simulink model "CSE1_HIL_full_Test"  (R2019b)
settings: Solver=VariableStepAuto  StartTime=0.0  StopTime=150  MaxStep=10e-3  RelTol=1e-3
values from neighbouring files (symbols this model uses):
  B = [zeros(3); inv(M); zeros(3)]    [CSE1_init.m]
  center_point = [0 0]'    [CSE1_init.m]
  D = [ ... (first row only)    [CSE1_init.m]    (also in D.m = reshape([abs(u).*(-3.545e-1)+u.^2.*3.787+6.555e-1,0.0,0.0,0.)
  end_point = [10 10]'    [CSE1_init.m]
  Kd = 1e-2    (= 0.01)    [CSE1_init.m]    (also in run.m = diag([40e-2 40e-2 40e-2]))
  Kp = 1e-2    (= 0.01)    [CSE1_init.m]    (also in run.m = diag([25e-2 25e-2 25e-4]))
  L1 = diag([1 1 1])    [CSE1_init.m]
  L2 = diag([0.1 0.1 0.1])    [CSE1_init.m]
  L3 = diag([0.025 0.01 0.0001])    [CSE1_init.m]
  M = [ ... (first row only)    [CSE1_init.m]
  measurement_signal_available = 1    [CSE1_init.m]
  measurment_noise = 0    [CSE1_init.m]
  my = 0.05    [CSE1_init.m]
  path_selection = 0    [CSE1_init.m]
  radius_xy = diag([1 2])    [CSE1_init.m]
  start_point = [0 0]'    [CSE1_init.m]
  U_ref = 0.15    [CSE1_init.m]
  x_init = zeros(1,9)    [CSE1_init.m]
libraries: simulink x1
settings Model: Creator=einarsu  LastModifiedBy=linnl
settings DataIOCC: ReturnWorkspaceOutputs=off
settings OptimizationCC: LifeSpan=inf
settings DebuggingCC: SFExecutionAtInitializationDiag=none  ArithmeticOperatorsInVariantConditions=warning
settings SFSimCC: SimUseLocalCustomCode=off  CustomCodeUndefinedFunction=UseInterfaceOnly
settings RTWCC: RTWUseLocalCustomCode=off
settings CodeAppCC: StateflowObjectComments=on

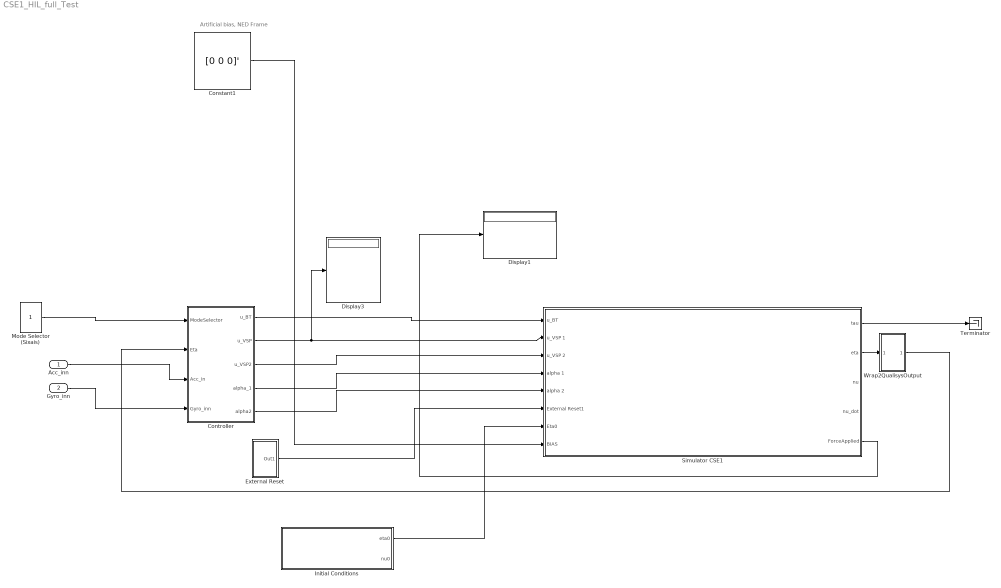
== system CSE1_HIL_full_Test ==
  note: Artificial bias, NED Frame
  Acc_inn : Inport
  Gyro_inn : Inport  Port=2
  Constant1 : Constant  Value=[0 0 0]'  VectorParams1D=off
  Controller : Subsystem
  Display1 : Display
  Display3 : Display
  External Reset : Subsystem
  "Initial Conditions " : Subsystem
  Mode Selector (Sixais) : Constant
  Simulator CSE1 : Subsystem
  Terminator : Terminator
  "Wrap2QualisysOutput " : Subsystem
  wires:
  Controller/1(u_BT) -> Simulator CSE1/1(u_BT)
  Controller/4(alpha_1) -> Simulator CSE1/4(alpha 1)
  Controller/2(u_VSP) -> Display3/1, Simulator CSE1/2(u_VSP 1)
  Controller/5(alpha2) -> Simulator CSE1/5(alpha 2)
  Controller/3("u_VSP2 ") -> Simulator CSE1/3(u_VSP 2)
  Simulator CSE1/1(tau) -> Terminator/1
  External Reset/1(Out1) -> Simulator CSE1/6(External Reset1)
  "Initial Conditions "/1(eta0) -> Simulator CSE1/7(Eta0)
  Mode Selector (Sixais)/1 -> Controller/1(ModeSelector)
  Simulator CSE1/2(eta) -> "Wrap2QualisysOutput "/1(In1)
  Acc_inn/1 -> Controller/3(Acc_in)
  Gyro_inn/1 -> Controller/4(Gyro_inn)
  Simulator CSE1/5(ForceApplied) -> Display1/1
  Constant1/1 -> Simulator CSE1/8(BIAS)
  "Wrap2QualisysOutput "/1(Out1) -> Controller/2(Eta)

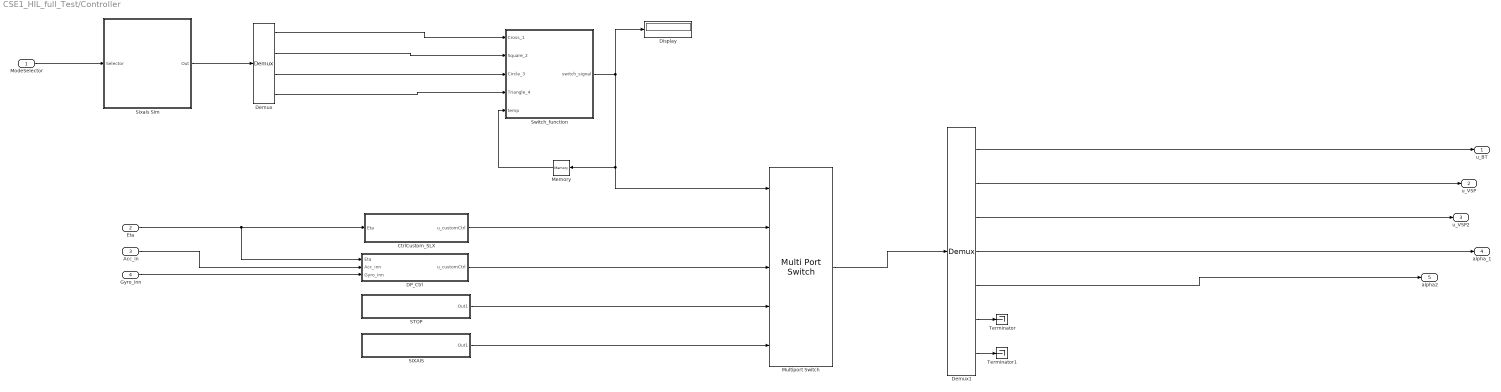
== system CSE1_HIL_full_Test/Controller ==
  ModeSelector : Inport
  Eta : Inport  Port=2
  Acc_in : Inport  Port=3
  Gyro_inn : Inport  Port=4
  CtrlCustom_SLX : Subsystem
  DP_Ctrl : Subsystem
  Demux : Demux
  Demux1 : Demux  Outputs=7
  Display : Display
  Memory : Memory  InitialCondition=4
  Multiport Switch : MultiPortSwitch  Inputs=4
  SIXAIS : Subsystem
  STOP : Subsystem
  Sixais Sim : MATLAB Function  TreatAsAtomicUnit=on
  Switch_function : MATLAB Function  TreatAsAtomicUnit=on
  Terminator : Terminator
  Terminator1 : Terminator
  u_BT : Outport
  u_VSP : Outport  Port=2
  "u_VSP2 " : Outport  Port=3
  alpha_1 : Outport  Port=4
  alpha2 : Outport  Port=5
  wires:
  Switch_function/1(switch_signal) -> Display/1, Memory/1, Multiport Switch/1
  Memory/1 -> Switch_function/5(temp)
  CtrlCustom_SLX/1(u_customCtrl) -> Multiport Switch/2
  Demux/1 -> Switch_function/1(Cross_1)
  Demux/2 -> Switch_function/2(Square_2)
  Demux/3 -> Switch_function/3(Circle_3)
  Demux/4 -> Switch_function/4(Triangle_4)
  Sixais Sim/1(Out) -> Demux/1
  ModeSelector/1 -> Sixais Sim/1(Selector)
  DP_Ctrl/1(u_customCtrl) -> Multiport Switch/3
  STOP/1(Out1) -> Multiport Switch/4
  SIXAIS/1(Out1) -> Multiport Switch/5
  Eta/1 -> CtrlCustom_SLX/1(Eta), DP_Ctrl/1(Eta)
  Acc_in/1 -> DP_Ctrl/2(Acc_inn)
  Gyro_inn/1 -> DP_Ctrl/3(Gyro_inn)
  Multiport Switch/1 -> Demux1/1
  Demux1/1 -> u_BT/1
  Demux1/2 -> u_VSP/1
  Demux1/3 -> "u_VSP2 "/1
  Demux1/4 -> alpha_1/1
  Demux1/5 -> alpha2/1
  Demux1/6 -> Terminator/1
  Demux1/7 -> Terminator1/1

== system CSE1_HIL_full_Test/External Reset ==
  note: Most relevant for Real-Time Simulations...
  Constant : Constant  Value=0
  Out1 : Outport
  wires:
  Constant/1 -> Out1/1

== system CSE1_HIL_full_Test/Initial Conditions  ==
  Eta0 : Constant  Value=zeros(3,1)
  "V0 " : Constant  Value=zeros(3,1)
  eta0 : Outport
  nu0 : Outport  Port=2
  wires:
  "V0 "/1 -> nu0/1
  Eta0/1 -> eta0/1

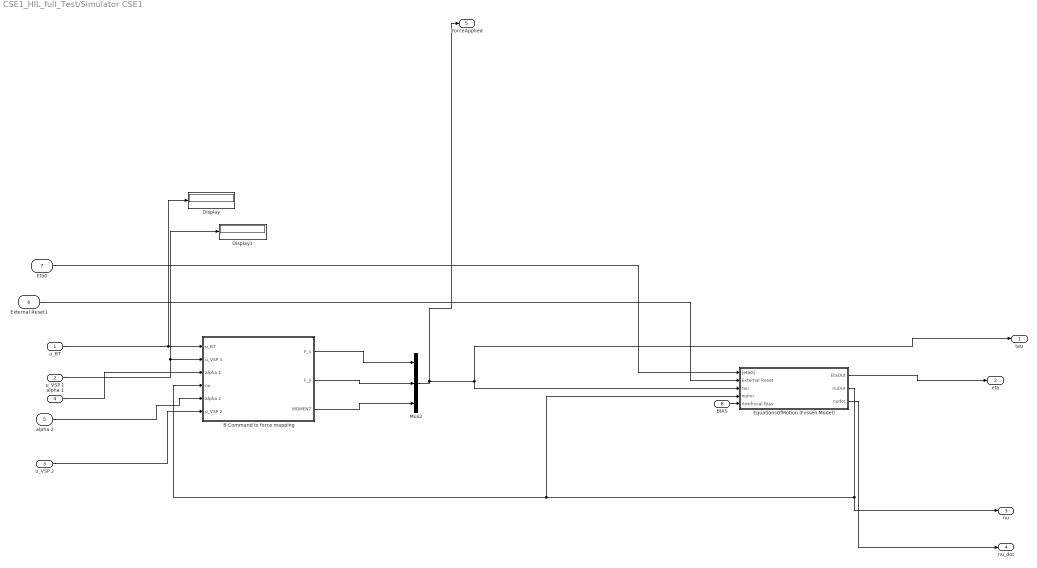
== system CSE1_HIL_full_Test/Simulator CSE1 ==
  u_BT : Inport
  u_VSP 1 : Inport  Port=2
  u_VSP 2 : Inport  Port=3
  alpha 1 : Inport  Port=4
  alpha 2 : Inport  Port=5
  External Reset1 : Inport  Port=6
  Eta0 : Inport  Port=7
  BIAS : Inport  Port=8
  B Command to force mapping : Subsystem
  Display : Display
  Display1 : Display
  EquationsOfMotion (Fossen Model) : Subsystem
  Mux2 : Mux  Inputs=3
  tau : Outport
  eta : Outport  Port=2
  nu : Outport  Port=3
  nu_dot : Outport  Port=4
  ForceApplied : Outport  Port=5
  wires:
  alpha 2/1 -> B Command to force mapping/5(alpha 2)
  B Command to force mapping/2("F_y ") -> Mux2/2
  B Command to force mapping/1(F_x) -> Mux2/1
  u_VSP 1/1 -> B Command to force mapping/2(u_VSP 1), Display1/1
  alpha 1/1 -> B Command to force mapping/3(alpha 1)
  u_BT/1 -> B Command to force mapping/1(u_BT), Display/1
  u_VSP 2/1 -> B Command to force mapping/6(u_VSP 2)
  EquationsOfMotion (Fossen Model)/2(nuOut) -> B Command to force mapping/4(nu), EquationsOfMotion (Fossen Model)/4(nuInn), nu/1
  Eta0/1 -> EquationsOfMotion (Fossen Model)/1("[eta0] ")
  External Reset1/1 -> EquationsOfMotion (Fossen Model)/2(External Reset)
  Mux2/1 -> ForceApplied/1, EquationsOfMotion (Fossen Model)/3(tau), tau/1
  EquationsOfMotion (Fossen Model)/1(EtaOut) -> eta/1
  EquationsOfMotion (Fossen Model)/3(nudot) -> nu_dot/1
  B Command to force mapping/3("MOMENT ") -> Mux2/3
  BIAS/1 -> EquationsOfMotion (Fossen Model)/5(Aritifiicial BIas)

== system CSE1_HIL_full_Test/Wrap2QualisysOutput  ==
  In1 : Inport
  Demux : Demux  Outputs=3
  Gain : Gain  Gain=1000
  Gain1 : Gain  Gain=1000
  Gain2 : Gain  Gain=180/pi
  Mux : Mux  Inputs=3
  Wrap2psi : MATLAB Function  TreatAsAtomicUnit=on
  Out1 : Outport
  wires:
  Mux/1 -> Out1/1
  In1/1 -> Demux/1
  Demux/3 -> Wrap2psi/1(u)
  Demux/1 -> Gain/1
  Demux/2 -> Gain1/1
  Gain/1 -> Mux/1
  Gain1/1 -> Mux/2
  Gain2/1 -> Mux/3
  Wrap2psi/1(yQualisus) -> Gain2/1

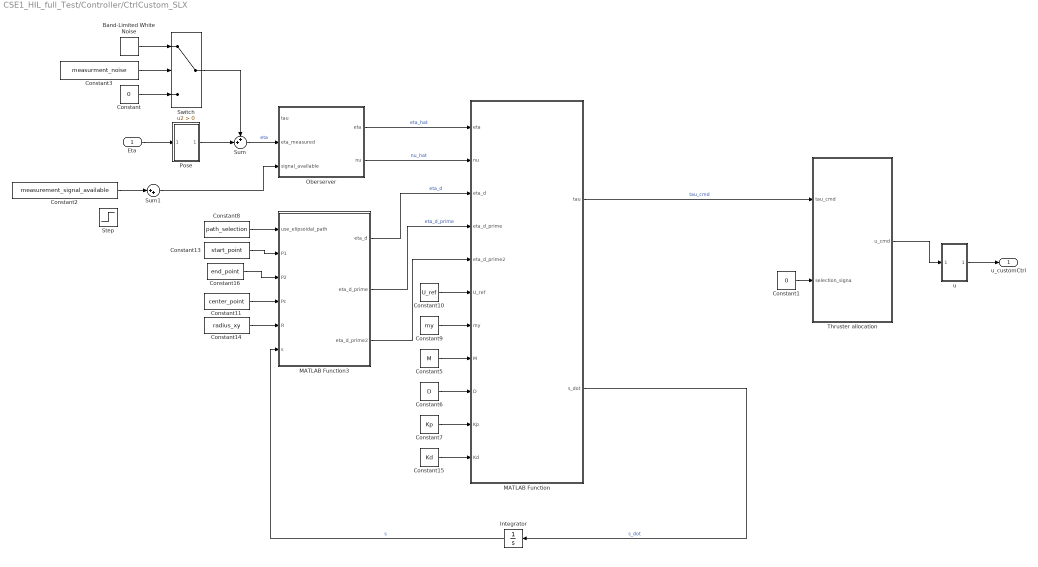
== system CSE1_HIL_full_Test/Controller/CtrlCustom_SLX ==
  Eta : Inport
  Band-Limited White Noise : simulink/Sources/Band-Limited White Noise  Cov=[0.01 0.01 0.001]'  Ts=0.1  seed=[23341]  VectorParams1D=off
  Constant : Constant  Value=0
  Constant1 : Constant  Value=0
  Constant10 : Constant  Value=U_ref
  Constant11 : Constant  Value=center_point
  Constant13 : Constant  Value=start_point
  Constant14 : Constant  Value=radius_xy
  Constant15 : Constant  Value=Kd
  Constant16 : Constant  Value=end_point
  Constant2 : Constant  Value=measurement_signal_available
  Constant3 : Constant  Value=measurment_noise
  Constant5 : Constant  Value=M
  Constant6 : Constant  Value=D
  Constant7 : Constant  Value=Kp
  Constant8 : Constant  Value=path_selection
  Constant9 : Constant  Value=my
  Integrator : Integrator
  MATLAB Function : MATLAB Function  TreatAsAtomicUnit=on
  MATLAB Function3 : MATLAB Function  TreatAsAtomicUnit=on
  Oberserver : Subsystem
  Pose : Subsystem
  Step : Step  Time=50  After=-1  SampleTime=0
  Sum : Sum  Inputs=++|
  Sum1 : Sum  Inputs=|++
  Switch : Switch  Criteria=u2 > Threshold
  Thruster allocation : Subsystem
  u : Subsystem
  u_customCtrl : Outport
  wires:
  Constant16/1 -> MATLAB Function3/3(P2)
  Constant14/1 -> MATLAB Function3/5(R)
  Constant15/1 -> MATLAB Function/11(Kd)
  Constant13/1 -> MATLAB Function3/2(P1)
  Oberserver/1(eta) -> MATLAB Function/1(eta)  "eta_hat"
  Eta/1 -> Pose/1(eta)
  Constant7/1 -> MATLAB Function/10(Kp)
  Thruster allocation/1(u_cmd) -> u/1(In1)
  Constant/1 -> Switch/3
  Constant1/1 -> Thruster allocation/2(selection_signa)
  u/1(Out1) -> u_customCtrl/1
  Constant10/1 -> MATLAB Function/6(U_ref)
  MATLAB Function3/3(eta_d_prime2) -> MATLAB Function/5(eta_d_prime2)
  Oberserver/2(nu) -> MATLAB Function/2(nu)  "nu_hat"
  MATLAB Function3/2(eta_d_prime) -> MATLAB Function/4(eta_d_prime)  "eta_d_prime"
  Sum1/1 -> Oberserver/3(signal_available)
  Constant9/1 -> MATLAB Function/7(my)
  Pose/1(QTM) -> Sum/2
  Constant2/1 -> Sum1/1
  MATLAB Function3/1(eta_d) -> MATLAB Function/3(eta_d)  "eta_d"
  Constant8/1 -> MATLAB Function3/1(use_elipsoidal_path)
  Band-Limited White Noise/1 -> Switch/1
  Sum/1 -> Oberserver/2(eta_measured)  "eta"
  Switch/1 -> Sum/1
  MATLAB Function/2(s_dot) -> Integrator/1  "s_dot"
  Constant11/1 -> MATLAB Function3/4(Pc)
  Constant5/1 -> MATLAB Function/8(M)
  Constant3/1 -> Switch/2
  Integrator/1 -> MATLAB Function3/6(s)  "s"
  MATLAB Function/1(tau) -> Thruster allocation/1(tau_cmd)  "tau_cmd"
  Constant6/1 -> MATLAB Function/9(D)

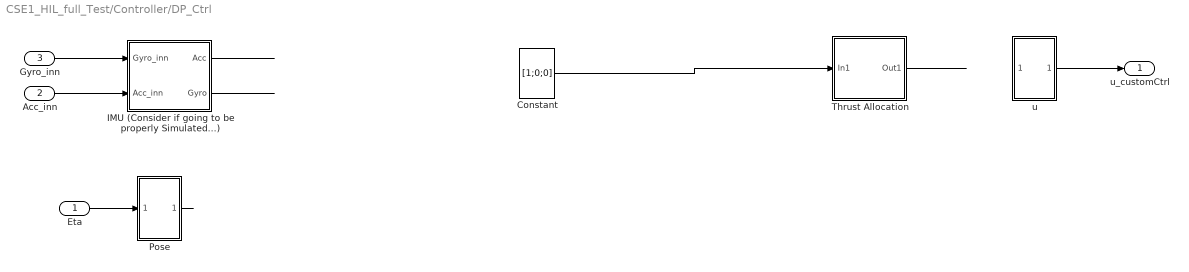
== system CSE1_HIL_full_Test/Controller/DP_Ctrl ==
  Eta : Inport
  Acc_inn : Inport  Port=2
  Gyro_inn : Inport  Port=3
  Constant : Constant  Value=[1;0;0]
  IMU (Consider if going to be properly Simulated...) : Subsystem
  Pose : Subsystem
  "Thrust Allocation " : Subsystem
  u : Subsystem
  u_customCtrl : Outport
  wires:
  Pose/1(QTM) -> ?
  Gyro_inn/1 -> IMU (Consider if going to be properly Simulated...)/1(Gyro_inn)
  Acc_inn/1 -> IMU (Consider if going to be properly Simulated...)/2(Acc_inn)
  Eta/1 -> Pose/1(eta)
  u/1(Out1) -> u_customCtrl/1
  IMU (Consider if going to be properly Simulated...)/2(Gyro) -> ?
  IMU (Consider if going to be properly Simulated...)/1(Acc) -> ?
  Constant/1 -> "Thrust Allocation "/1(In1)
  "Thrust Allocation "/1(Out1) -> ?

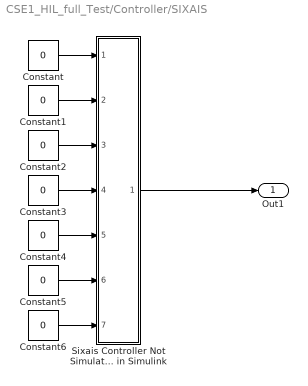
== system CSE1_HIL_full_Test/Controller/SIXAIS ==
  Constant{,1..6} (7 alike) : Constant  Value=0
  Sixais Controller Not Simulated in Simulink : Subsystem
  Out1 : Outport
  wires:
  Constant/1 -> Sixais Controller Not Simulated in Simulink/1(In1)
  Constant1/1 -> Sixais Controller Not Simulated in Simulink/2(In2)
  Constant2/1 -> Sixais Controller Not Simulated in Simulink/3(In3)
  Constant3/1 -> Sixais Controller Not Simulated in Simulink/4(In4)
  Constant4/1 -> Sixais Controller Not Simulated in Simulink/5(In5)
  Constant5/1 -> Sixais Controller Not Simulated in Simulink/6(In6)
  Constant6/1 -> Sixais Controller Not Simulated in Simulink/7(In7)
  Sixais Controller Not Simulated in Simulink/1(Out1) -> Out1/1

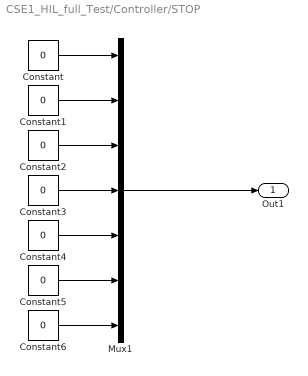
== system CSE1_HIL_full_Test/Controller/STOP ==
  Constant{,1..6} (7 alike) : Constant  Value=0
  Mux1 : Mux  Inputs=7
  Out1 : Outport
  wires:
  Mux1/1 -> Out1/1
  Constant/1 -> Mux1/1
  Constant1/1 -> Mux1/2
  Constant2/1 -> Mux1/3
  Constant3/1 -> Mux1/4
  Constant4/1 -> Mux1/5
  Constant5/1 -> Mux1/6
  Constant6/1 -> Mux1/7

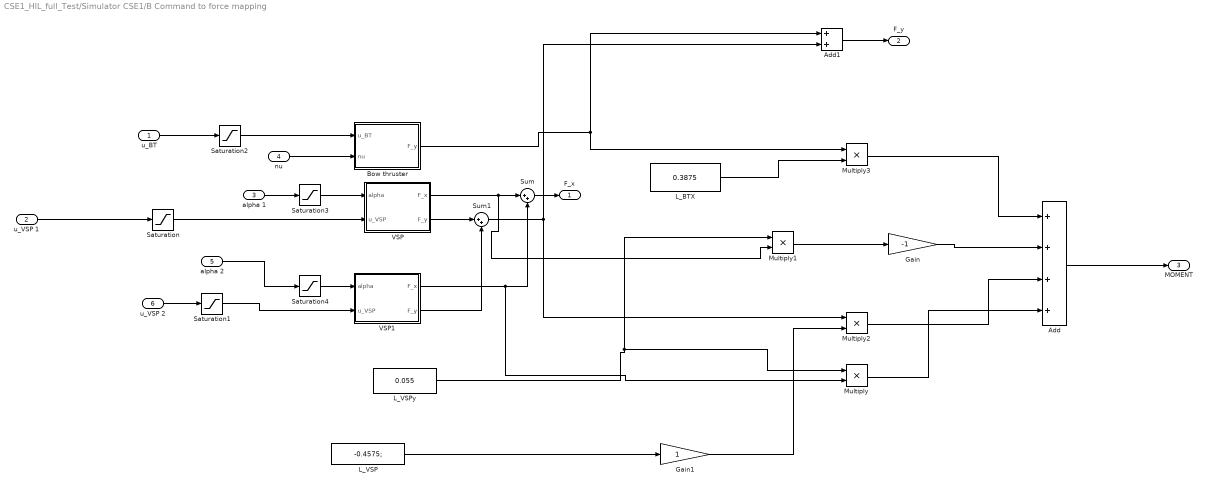
== system CSE1_HIL_full_Test/Simulator CSE1/B Command to force mapping ==
  u_BT : Inport
  u_VSP 1 : Inport  Port=2
  alpha 1 : Inport  Port=3
  nu : Inport  Port=4
  alpha 2 : Inport  Port=5
  u_VSP 2 : Inport  Port=6
  Add : Sum  Inputs=++++
  Add1 : Sum
  Bow thruster : MATLAB Function  TreatAsAtomicUnit=on
  Gain : Gain  Gain=-1
  Gain1 : Gain
  L_BTX : Constant  Value=0.3875
  L_VSP : Constant  Value=-0.4575;
  L_VSPy : Constant  Value=0.055
  Multiply{,1..3} (4 alike) : Product
  Saturation : Saturate  UpperLimit=1  LowerLimit=0
  Saturation1 : Saturate  UpperLimit=1  LowerLimit=0
  Saturation2 : Saturate  UpperLimit=1  LowerLimit=-1
  Saturation3 : Saturate  UpperLimit=pi  LowerLimit=-pi
  Saturation4 : Saturate  UpperLimit=pi  LowerLimit=-pi
  Sum : Sum  Inputs=|++
  Sum1 : Sum  Inputs=|++
  VSP : MATLAB Function  TreatAsAtomicUnit=on
  VSP1 : MATLAB Function  TreatAsAtomicUnit=on
  F_x : Outport
  "F_y " : Outport  Port=2
  "MOMENT " : Outport  Port=3
  wires:
  alpha 1/1 -> Saturation3/1
  nu/1 -> Bow thruster/2(nu)
  Bow thruster/1(F_y) -> Add1/1, Multiply3/1
  VSP/2(F_y) -> Sum1/1
  Sum1/1 -> Add1/2, Multiply2/1
  VSP1/2(F_y) -> Sum1/2
  VSP1/1(F_x) -> Multiply/2, Sum/2
  VSP/1(F_x) -> Multiply1/2, Sum/1
  Sum/1 -> F_x/1
  alpha 2/1 -> Saturation4/1
  u_VSP 2/1 -> Saturation1/1
  L_VSP/1 -> Gain1/1
  L_BTX/1 -> Multiply3/2
  L_VSPy/1 -> Multiply/1, Multiply1/1
  Multiply3/1 -> Add/1
  Multiply1/1 -> Gain/1
  Multiply2/1 -> Add/3
  Multiply/1 -> Add/4
  Add/1 -> "MOMENT "/1
  Gain/1 -> Add/2
  Gain1/1 -> Multiply2/2
  Add1/1 -> "F_y "/1
  Saturation/1 -> VSP/2(u_VSP)
  Saturation1/1 -> VSP1/2(u_VSP)
  u_BT/1 -> Saturation2/1
  u_VSP 1/1 -> Saturation/1
  Saturation2/1 -> Bow thruster/1(u_BT)
  Saturation3/1 -> VSP/1(alpha)
  Saturation4/1 -> VSP1/1(alpha)

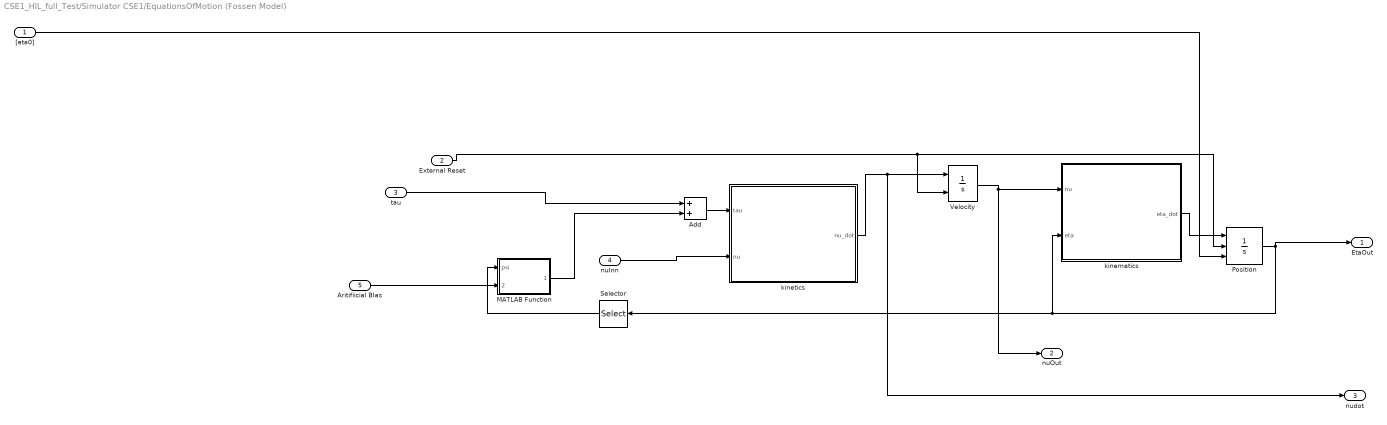
== system CSE1_HIL_full_Test/Simulator CSE1/EquationsOfMotion (Fossen Model) ==
  "[eta0] " : Inport
  External Reset : Inport  Port=2
  tau : Inport  Port=3
  nuInn : Inport  Port=4
  Aritifiicial BIas : Inport  Port=5
  Add : Sum
  MATLAB Function : MATLAB Function  TreatAsAtomicUnit=on
  Position : Integrator  ExternalReset=either  InitialConditionSource=external  InitialCondition=[0 0 0]'
  Selector : Selector  InputPortWidth=3  IndexOptions=Index vector (dialog)  Indices=[3]  OutputSizes=1
  Velocity : Integrator  ExternalReset=either  InitialCondition=[0 0 0]'
  kinematics : MATLAB Function  TreatAsAtomicUnit=on
  kinetics : MATLAB Function  TreatAsAtomicUnit=on
  EtaOut : Outport
  nuOut : Outport  Port=2
  nudot : Outport  Port=3
  wires:
  tau/1 -> Add/1
  Position/1 -> Selector/1, kinematics/2(eta), EtaOut/1
  "[eta0] "/1 -> Position/3
  nuInn/1 -> kinetics/2(nu)
  kinematics/1(eta_dot) -> Position/1
  Velocity/1 -> nuOut/1, kinematics/1(nu)
  kinetics/1(nu_dot) -> nudot/1, Velocity/1
  External Reset/1 -> Velocity/2, Position/2
  Add/1 -> kinetics/1(tau)
  Aritifiicial BIas/1 -> MATLAB Function/2(NedVector)
  Selector/1 -> MATLAB Function/1(psi)
  MATLAB Function/1(BodyVector) -> Add/2

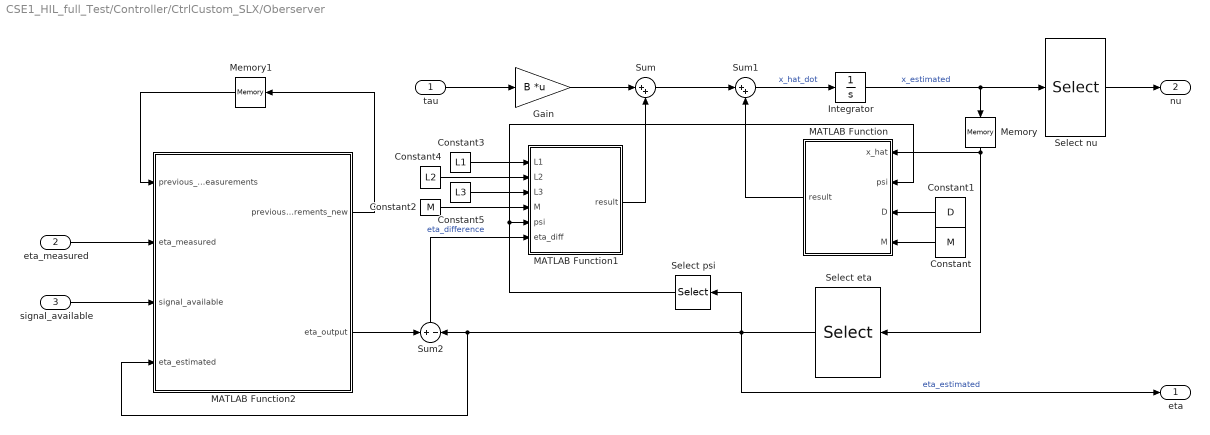
== system CSE1_HIL_full_Test/Controller/CtrlCustom_SLX/Oberserver ==
  tau : Inport
  eta_measured : Inport  Port=2
  signal_available : Inport  Port=3
  Constant : Constant  Value=M
  Constant1 : Constant  Value=D
  Constant2 : Constant  Value=M
  Constant3 : Constant  Value=L1
  Constant4 : Constant  Value=L2
  Constant5 : Constant  Value=L3
  Gain : Gain  Gain=B  Multiplication=Matrix(K*u) (u vector)
  Integrator : Integrator  InitialCondition=x_init
  MATLAB Function : MATLAB Function  TreatAsAtomicUnit=on
  MATLAB Function1 : MATLAB Function  TreatAsAtomicUnit=on
  MATLAB Function2 : MATLAB Function  TreatAsAtomicUnit=on
  Memory : Memory  InitialCondition=x_init
  Memory1 : Memory  InitialCondition=[0,0,0; 0,0,0; 0,0,0]
  Select eta : Selector  InputPortWidth=9  IndexOptions=Index vector (dialog)  Indices=[1 2 3]  OutputSizes=1
  Select nu : Selector  InputPortWidth=9  IndexOptions=Index vector (dialog)  Indices=[4 5 6]  OutputSizes=1
  Select psi : Selector  InputPortWidth=3  IndexOptions=Index vector (dialog)  Indices=[3]  OutputSizes=1
  Sum : Sum  Inputs=|++
  Sum1 : Sum  Inputs=|++
  Sum2 : Sum  Inputs=+|-
  eta : Outport
  nu : Outport  Port=2
  wires:
  Integrator/1 -> Select nu/1, Memory/1  "x_estimated"
  tau/1 -> Gain/1
  Gain/1 -> Sum/1
  Sum1/1 -> Integrator/1  "x_hat_dot"
  Sum/1 -> Sum1/1
  eta_measured/1 -> MATLAB Function2/2(eta_measured)
  MATLAB Function1/1(result) -> Sum/2
  MATLAB Function/1(result) -> Sum1/2
  Constant/1 -> MATLAB Function/4(M)
  Constant1/1 -> MATLAB Function/3(D)
  Memory/1 -> Select eta/1, MATLAB Function/1(x_hat)
  Select eta/1 -> MATLAB Function2/4(eta_estimated), Sum2/2, Select psi/1, eta/1  "eta_estimated"
  Constant2/1 -> MATLAB Function1/4(M)
  Constant3/1 -> MATLAB Function1/1(L1)
  Constant4/1 -> MATLAB Function1/2(L2)
  Constant5/1 -> MATLAB Function1/3(L3)
  signal_available/1 -> MATLAB Function2/3(signal_available)
  MATLAB Function2/1(previous_measurements_new) -> Memory1/1
  Memory1/1 -> MATLAB Function2/1(previous_measurements)
  Select nu/1 -> nu/1
  MATLAB Function2/2(eta_output) -> Sum2/1
  Sum2/1 -> MATLAB Function1/6(eta_diff)  "eta_difference"
  Select psi/1 -> MATLAB Function/2(psi), MATLAB Function1/5(psi)

== system CSE1_HIL_full_Test/Controller/CtrlCustom_SLX/Pose ==
  eta : Inport
  Demux : Demux  Outputs=3
  Gain : Gain  Gain=10^-3
  Gain1 : Gain  Gain=10^-3
  MATLAB Function : MATLAB Function  TreatAsAtomicUnit=on
  Mux : Mux  Inputs=3
  QTM : Outport
  wires:
  Demux/2 -> Gain1/1  "y_mm"
  Demux/3 -> MATLAB Function/1(deg)  "psi_deg"
  Mux/1 -> QTM/1
  eta/1 -> Demux/1
  Demux/1 -> Gain/1  "x_mm"
  Gain/1 -> Mux/1  "x_m"
  Gain1/1 -> Mux/2  "y_m"
  MATLAB Function/1(rad) -> Mux/3  "psi_rad"

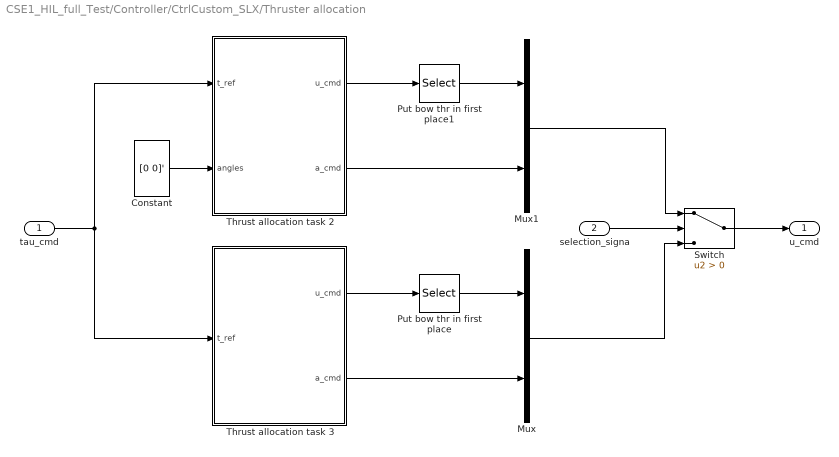
== system CSE1_HIL_full_Test/Controller/CtrlCustom_SLX/Thruster allocation ==
  tau_cmd : Inport
  selection_signa : Inport  Port=2
  Constant : Constant  Value=[0 0]'  VectorParams1D=off
  Mux : Mux  Inputs=2
  Mux1 : Mux  Inputs=2
  Put bow thr in first place : Selector  InputPortWidth=3  IndexOptions=Index vector (dialog)  Indices=[3 1 2]  OutputSizes=1
  Put bow thr in first place1 : Selector  InputPortWidth=3  IndexOptions=Index vector (dialog)  Indices=[3 1 2]  OutputSizes=1
  Switch : Switch  Criteria=u2 > Threshold
  Thrust allocation task 2 : Subsystem
  Thrust allocation task 3 : Subsystem
  u_cmd : Outport
  wires:
  Switch/1 -> u_cmd/1
  Constant/1 -> Thrust allocation task 2/2(angles)
  Thrust allocation task 2/1(u_cmd) -> Put bow thr in first place1/1
  Thrust allocation task 2/2(a_cmd) -> Mux1/2
  Put bow thr in first place1/1 -> Mux1/1
  Mux1/1 -> Switch/1
  Thrust allocation task 3/2(a_cmd) -> Mux/2
  Thrust allocation task 3/1(u_cmd) -> Put bow thr in first place/1
  Put bow thr in first place/1 -> Mux/1
  Mux/1 -> Switch/3
  selection_signa/1 -> Switch/2
  tau_cmd/1 -> Thrust allocation task 3/1(t_ref), Thrust allocation task 2/1(t_ref)

== system CSE1_HIL_full_Test/Controller/CtrlCustom_SLX/u ==
  In1 : Inport
  Constant : Constant  Value=0.3
  Constant1 : Constant  Value=0.3
  Demux1 : Demux  Outputs=5
  Mux : Mux  Inputs=7
  Saturation1 : Saturate  UpperLimit=1  LowerLimit=0
  Saturation11 : Saturate  UpperLimit=1  LowerLimit=0
  Out1 : Outport
  wires:
  In1/1 -> Demux1/1
  Demux1/1 -> Mux/1  "u_BT"
  Demux1/2 -> Saturation11/1  "u_VSP1"
  Demux1/3 -> Saturation1/1  "u_VSP2"
  Demux1/4 -> Mux/4  "alpha_VSP1"
  Demux1/5 -> Mux/5  "alpha_VSP2"
  Constant/1 -> Mux/6  "omega_VSP1"
  Constant1/1 -> Mux/7  "omega_VSP2"
  Mux/1 -> Out1/1
  Saturation11/1 -> Mux/2
  Saturation1/1 -> Mux/3

== system CSE1_HIL_full_Test/Controller/DP_Ctrl/IMU (Consider if going to be properly Simulated...) ==
  Gyro_inn : Inport
  Acc_inn : Inport  Port=2
  Demux : Demux  Outputs=3
  Demux1 : Demux  Outputs=3
  Mux : Mux  Inputs=3
  Mux2 : Mux  Inputs=3
  Acc : Outport
  Gyro : Outport  Port=2
  wires:
  Acc_inn/1 -> Demux1/1
  Gyro_inn/1 -> Demux/1
  Demux/1 -> Mux2/1
  Demux/2 -> Mux2/2
  Demux/3 -> Mux2/3
  Demux1/2 -> Mux/2
  Demux1/3 -> Mux/3
  Mux2/1 -> Gyro/1
  Demux1/1 -> Mux/1
  Mux/1 -> Acc/1

== system CSE1_HIL_full_Test/Controller/DP_Ctrl/Pose ==
  eta : Inport
  Demux : Demux  Outputs=3
  Mux : Mux  Inputs=3
  QTM : Outport
  wires:
  eta/1 -> Demux/1
  Mux/1 -> QTM/1
  Demux/1 -> Mux/1  "x_m"
  Demux/3 -> Mux/3  "psi_m"
  Demux/2 -> Mux/2  "y_m"

== system CSE1_HIL_full_Test/Controller/DP_Ctrl/Thrust Allocation  ==
  In1 : Inport
  THALOC (u->tau) : MATLAB Function  TreatAsAtomicUnit=on
  Out1 : Outport
  wires:
  In1/1 -> THALOC (u->tau)/1(u)
  THALOC (u->tau)/1(y) -> Out1/1

== system CSE1_HIL_full_Test/Controller/DP_Ctrl/u ==
  In1 : Inport
  Demux1 : Demux  Outputs=7
  Mux : Mux  Inputs=7
  Out1 : Outport
  wires:
  Mux/1 -> Out1/1
  Demux1/7 -> Mux/7  "omega_VSP2"
  Demux1/6 -> Mux/6  "omega_VSP1"
  Demux1/5 -> Mux/5  "alpha_VSP2"
  Demux1/4 -> Mux/4  "alpha_VSP1"
  Demux1/3 -> Mux/3  "u_VSP2"
  Demux1/2 -> Mux/2  "u_VSP1"
  Demux1/1 -> Mux/1  "u_BT"
  In1/1 -> Demux1/1

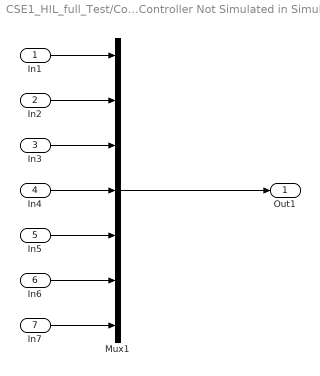
== system CSE1_HIL_full_Test/Controller/SIXAIS/Sixais Controller Not Simulated in Simulink ==
  In1 : Inport
  In2 : Inport  Port=2
  In3 : Inport  Port=3
  In4 : Inport  Port=4
  In5 : Inport  Port=5
  In6 : Inport  Port=6
  In7 : Inport  Port=7
  Mux1 : Mux  Inputs=7
  Out1 : Outport
  wires:
  In4/1 -> Mux1/4
  In5/1 -> Mux1/5
  In6/1 -> Mux1/6
  In3/1 -> Mux1/3
  In1/1 -> Mux1/1
  In2/1 -> Mux1/2
  Mux1/1 -> Out1/1
  In7/1 -> Mux1/7

== system CSE1_HIL_full_Test/Controller/CtrlCustom_SLX/Thruster allocation/Thrust allocation task 2 ==
  t_ref : Inport
  angles : Inport  Port=2
  MATLAB Function : MATLAB Function  TreatAsAtomicUnit=on
  MATLAB Function1 : MATLAB Function  TreatAsAtomicUnit=on
  u_cmd : Outport
  a_cmd : Outport  Port=2
  wires:
  MATLAB Function1/2(a_cmd) -> a_cmd/1
  MATLAB Function1/1(u_cmd) -> u_cmd/1
  t_ref/1 -> MATLAB Function/1(t_ref)
  MATLAB Function/1(u_star) -> MATLAB Function1/1(u_star)
  angles/1 -> MATLAB Function1/2(a), MATLAB Function/2(angles)

== system CSE1_HIL_full_Test/Controller/CtrlCustom_SLX/Thruster allocation/Thrust allocation task 3 ==
  t_ref : Inport
  MATLAB Function : MATLAB Function  TreatAsAtomicUnit=on
  MATLAB Function1 : MATLAB Function  TreatAsAtomicUnit=on
  u_cmd : Outport
  a_cmd : Outport  Port=2
  wires:
  MATLAB Function1/2(a_cmd) -> a_cmd/1
  MATLAB Function1/1(u_cmd) -> u_cmd/1
  MATLAB Function/1(u_star) -> MATLAB Function1/1(u_star)
  t_ref/1 -> MATLAB Function/1(t_ref)

== matlab function CSE1_HIL_full_Test/Simulator CSE1/EquationsOfMotion (Fossen Model)/kinematics ==
  data: nu input; eta_dot output; eta input
function eta_dot = CSE1_eta_dot(nu,eta)

psi = eta(3);

J = [cos(psi) -sin(psi) 0
     sin(psi) cos(psi)  0
     0        0         1];

eta_dot = J*nu;

== matlab function CSE1_HIL_full_Test/Simulator CSE1/EquationsOfMotion (Fossen Model)/kinetics ==
  data: tau input; nu_dot output; nu input
function nu_dot = CSE1_nu_dot(tau,nu)

u   = nu(1);
v   = nu(2);
r   = nu(3);

tau = [tau(1);tau(2);tau(3)];
%% MATRICES 
%changed m from 14.79 to 14.11

m    = 14.11;   I_z  =  1.7600;   x_g = 0.0375;       % x_g  =  0.0460; % Table B.1

%% Added mass
%changed Y_vd from -1.0 to -10.0
X_ud  =     -2.0;											% Table B.1
					Y_vd =      -10.0;	N_vd =    -0.0;		% Table B.1
					Y_rd =      -0.0;	N_rd =    -1.0;		% Table B.1

%% Total mass matrix
m_11 = m-X_ud;
m_22 = m-Y_vd;
m_23 = m*x_g-Y_rd;
m_32 = m*x_g-N_vd; % noted as Y_rd in handbook, but same value
m_33 = I_z-N_rd;

M    = [m_11 0    0
        0    m_22 m_23
        0    m_32 m_33];
	
%% Damping coefficients
% Comments at the end of the lines indicate the old values used.
X_u		= -0.6555;		X_v		= 0;
X_uu 	= 0.3545;		X_vv	= -2.443;
X_uuu 	= -3.787;		X_vvv	= 0;

						Y_v		= -1.33; 			Y_r		= -7.250; % Y_r
						Y_vv	= -2.776;			Y_rr	= -3.450; % Y_rr
						Y_vvv	= -64.91;			Y_rrr	= 0;
						
						Y_rv	= -0.805;			Y_vr	= -0.845; % Y_rv, Y_vr

						N_v		= 0;				N_r		= -1.900; % N_r
						N_vv	= -0.2088;			N_rr	= -0.750; % N_rr
						N_vvv	= 0;				N_rrr	= 0;
						
						N_rv	= 0.130;			N_vr	= 0.080; % N_rv, N_vr

%% Correolis matrix
c_13 = -(m-Y_vd)*v-(m*x_g-Y_rd)*r;
c_23 = (m-X_ud)*u;
C    = [0     0     c_13
        0     0     c_23
        -c_13 -c_23 0   ];

%% Assembly of the damping matrix
%should be abs(u), abs(v) some places, only positive values? 

d_11 = -X_u - X_uu*u - X_uuu*u^2;
d_22 = -Y_v - Y_vv*v - Y_vvv*v^2 - Y_rv*abs(r);
d_33 = -N_r - N_rr*abs(r) - N_rrr*r^2 - N_vr*abs(v); % using abs(r)

d_12 = -X_v - X_vv*v - X_vvv*v^2;
d_23 = -Y_r - Y_rr*abs(r) - Y_rrr*r^2 - Y_vr*abs(v);
d_32 = -N_v - N_vv*v - N_vvv*v^2 - N_rv*abs(r);

%D    = [d_11 d_12 0      vet ikke hvorfor d_12 er her
%        0    d_22 d_23
%        0    d_32 d_33];
D    = [d_11 0 0
        0    d_22 d_23
        0    d_32 d_33];


%% CALCULATION
nu_dot = M\(tau-(C+D)*nu);

== matlab function CSE1_HIL_full_Test/Simulator CSE1/EquationsOfMotion (Fossen Model)/MATLAB Function ==
  data: psi input; BodyVector output; NedVector input
function BodyVector = fcn(psi,NedVector)
R=[cos(psi) sin(psi) 0; -sin(psi) cos(psi) 0;0 0 1];
BodyVector=R*NedVector;
end

== matlab function CSE1_HIL_full_Test/Wrap2QualisysOutput /Wrap2psi ==
  data: u input; yQualisus output
function yQualisus = fcn(u)
y=sin(u)
x=cos(u)
yQualisus=atan2(y,x);
end

== matlab function CSE1_HIL_full_Test/Controller/CtrlCustom_SLX/Thruster allocation/Thrust allocation task 2/MATLAB Function ==
  data: t_ref input; u_star output; angles input
function u_star = thrust_allocation_2(t_ref, angles)
% Calculates thrust and vsp angles for set angles

% Parameters
lx_1 = 0.3875;
lx_2 = -0.4574;
ly_1 = 0.055;
ly_2 = -0.055;

K1 = 1.03;
K2 = K1;
K3 = 2.629;

a1 = angles(1);
a2 = angles(2);

B = [cos(a1) cos(a2) 0; 
    sin(a1) sin(a2) 1; 
    lx_2*sin(a1)-ly_1*cos(a2) lx_2*sin(a2)-ly_2*cos(a2) lx_1];
K = diag([K1, K2, K3]);

% Calculate u with pseudo inverse method
u_star = pinv(B*K) * t_ref;

end

== matlab function CSE1_HIL_full_Test/Controller/CtrlCustom_SLX/Thruster allocation/Thrust allocation task 2/MATLAB Function1 ==
  data: u_star input; u_cmd output; a input; a_cmd output
function [u_cmd, a_cmd] = beta_procedure(u_star, a)
% Flips angle and thrust if thrust is negative

% initialize outputs
u_cmd = [0 0 0]';
a_cmd = [0 0]';

if u_star(1) < 0
    % flip thrust
    u_cmd(1) = - u_star(1);
    
    % flip angle
    if a(1) < 0
        a_cmd(1) = a(1) + pi;
    else
        a_cmd(1) = a(1) - pi;
    end
else
    a_cmd(1) = a(1);
    u_cmd(1) = u_star(1);
end
    
if u_star(2) < 0
    % flip thrust
    u_cmd(2) = - u_star(2);
    
    % flip angle
    if a(2) < 0
        a_cmd(2) = a(2) + pi;
    else
        a_cmd(2) = a(2) - pi;
    end
else
    a_cmd(2) = a(2);
    u_cmd(2) = u_star(2);
end

u_cmd(3) = u_star(3);
    
end

== matlab function CSE1_HIL_full_Test/Controller/CtrlCustom_SLX/Thruster allocation/Thrust allocation task 3/MATLAB Function ==
  data: t_ref input; u_star output
function u_star = thrust_allocation_3(t_ref)

% parameters
lx_1 = 0.3875;
lx_2 = -0.4574;
ly_1 = 0.055;
ly_2 = -0.055;

K1 = 1.03;
K2 = K1;
K3 = 2.629;

K = diag([K1, K1, K2, K2, K3]);
B = [
    1 0 1 0 0;
    0 1 0 1 1;
    ly_1 lx_2 ly_2 lx_2 lx_1;
];

% Calculate thrust cmd using pseude inverse method
u_star = pinv(B*K)*t_ref;

end

== matlab function CSE1_HIL_full_Test/Controller/Switch_function ==
  data: Cross_1 input; switch_signal output; Square_2 input; Circle_3 input; Triangle_4 input; temp input
%% Function that takes in impulse button sigals [0,1] and sends out a 
% different signal depentent pn which button has been pressed

function switch_signal = fcn(Cross_1,Square_2,Circle_3,Triangle_4,temp)
%#codegen
persistent signal;

signal = temp;

if Cross_1 ~= 0
    signal = 1;
end

if Square_2 ~= 0
    signal = 2;
end

if Circle_3 ~= 0
    signal = 3;
end
    
if Triangle_4 ~= 0
    signal = 4; 
end

switch_signal = signal;

== matlab function CSE1_HIL_full_Test/Controller/Sixais Sim ==
  data: Selector input; Out output
%% Function that takes in impulse button sigals [0,1] and sends out a 
% different signal depentent pn which button has been pressed

function Out = fcn(Selector)
%#codegen
if Selector==1
    Out=[1 0 0 0];
elseif Selector==2
        Out=[0 1 0 0];
elseif Selector==4
        Out=[0 0 0 1];
else 
        Out=[0 0 1 0];

end

== matlab function CSE1_HIL_full_Test/Controller/DP_Ctrl/Thrust Allocation /THALOC (u->tau) ==
  data: u input; y output
function y = fcn(u)

y = u;

== matlab function CSE1_HIL_full_Test/Controller/CtrlCustom_SLX/Thruster allocation/Thrust allocation task 3/MATLAB Function1 ==
  data: u_star input; u_cmd output; a_cmd output
function [u_cmd, a_cmd] = gamma_procedure(u_star)
% param u_decomposed = [u1_x, u1_y, u2_x, u2_y, u3]
% this function maps u_decomposed to its thruster input and angles

% TODO: limit output u to [0,1]?

% initialize output values
u_cmd = [0 0 0]';
a_cmd = [0 0]';

u1_x = u_star(1);
u1_y = u_star(2);
u2_x = u_star(3);
u2_y = u_star(4);
u_cmd(3) = u_star(5);

a_cmd(1) = atan2(u1_y, u1_x);
a_cmd(2) = atan2(u2_y, u2_x);

u_cmd(1) = norm([u1_x, u1_y]);
u_cmd(2) = norm([u2_x, u2_y]);

end

== matlab function CSE1_HIL_full_Test/Simulator CSE1/B Command to force mapping/Bow thruster ==
  data: u_BT input; F_y output; nu input
function F_y = fcn(u_BT,nu)
%#codegen
u = nu(1);
% Thruster characteristics
if u_BT >0
    u_BT=u_BT+ 0.059;
    a =        -548;
    b =       0.193;
    c =       548.2;
    d =      0.1992;
    y0 = -(a*exp(b*-u_BT) + c*exp(d*-u_BT));
elseif u_BT < 0
    u_BT=u_BT- 0.059;
    a =        -548;
    b =       0.193;
    c =       548.2;
    d =      0.1992;
    y0 = a*exp(b*u_BT) + c*exp(d*u_BT);
else
    y0 = 0;
end
% Thruster losses due to forward speed
a0 =      0.7561;
a1 =      0.3075;
b1 =      -10.22;
c1 =       2.947;
F_y = y0*(a0 + a1*atan(b1*u +c1))/1.1385;
F_y=F_y*2.62/2.7629;


%2019 changes- Some add-hock changes, because it did not make sense previously.

== matlab function CSE1_HIL_full_Test/Simulator CSE1/B Command to force mapping/VSP ==
  data: alpha input; F_x output; u_VSP input; F_y output
function [ F_x , F_y ] = fcn(alpha,u_VSP)
%#codegen
% Calculating the force in x-direction
a1 =       1.107  ;
b1 =       1.001  ;
c1 =       1.564  ;
a2 =      0.3471 ;
b2 =      0.1397 ;
c2 =      -1.599  ;
a3 =      0.1558 ;
b3 =       1.993  ;
c3 =       1.886  ;
a4 =      0.1599 ;
b4 =       0.218  ;
c4 =       1.513  ;
a5 =     0.08237 ;
b5 =       2.986  ;
c5 =      -1.601  ;
a6 =     0.04641 ;
b6 =       3.964  ;
c6 =       1.738  ;
F_x =   u_VSP*( a1*sin(b1*alpha+c1) + ...
                a2*sin(b2*alpha+c2) + ...
                a3*sin(b3*alpha+c3) + ...
                a4*sin(b4*alpha+c4) + ...
                a5*sin(b5*alpha+c5) + ...
                a6*sin(b6*alpha+c6) );
% Calculating the force in y-direction
a1 =      0.7936 ;
b1 =       1.001  ;
c1 =     0.01605;
a2 =      0.2112 ;
b2 =       1.997  ;
c2 =     0.03229;
a3 =     0.07608;
b3 =       2.991  ;
c3 =       2.986  ;
a4 =     0.04817;
b4 =       3.999  ;
c4 =     -0.8668 ;
a5 =     0.01757;
b5 =       4.904  ;
c5 =      -2.622 ;
a6 =    -0.02089;
b6 =       5.068  ;
c6 =      0.2548 ;
F_y =   u_VSP*( a1*sin(b1*alpha+c1) + ...
                a2*sin(b2*alpha+c2) + ...
                a3*sin(b3*alpha+c3) + ...
                a4*sin(b4*alpha+c4) + ...
                a5*sin(b5*alpha+c5) + ...
                a6*sin(b6*alpha+c6));

== matlab function CSE1_HIL_full_Test/Simulator CSE1/B Command to force mapping/VSP1 ==
  data: alpha input; F_x output; u_VSP input; F_y output
function [ F_x , F_y ] = fcn(alpha,u_VSP)
%#codegen
% Calculating the force in x-direction
a1 =       1.107  ;
b1 =       1.001  ;
c1 =       1.564  ;
a2 =      0.3471 ;
b2 =      0.1397 ;
c2 =      -1.599  ;
a3 =      0.1558 ;
b3 =       1.993  ;
c3 =       1.886  ;
a4 =      0.1599 ;
b4 =       0.218  ;
c4 =       1.513  ;
a5 =     0.08237 ;
b5 =       2.986  ;
c5 =      -1.601  ;
a6 =     0.04641 ;
b6 =       3.964  ;
c6 =       1.738  ;
F_x =   u_VSP*( a1*sin(b1*alpha+c1) + ...
                a2*sin(b2*alpha+c2) + ...
                a3*sin(b3*alpha+c3) + ...
                a4*sin(b4*alpha+c4) + ...
                a5*sin(b5*alpha+c5) + ...
                a6*sin(b6*alpha+c6) );
% Calculating the force in y-direction
a1 =      0.7936 ;
b1 =       1.001  ;
c1 =     0.01605;
a2 =      0.2112 ;
b2 =       1.997  ;
c2 =     0.03229;
a3 =     0.07608;
b3 =       2.991  ;
c3 =       2.986  ;
a4 =     0.04817;
b4 =       3.999  ;
c4 =     -0.8668 ;
a5 =     0.01757;
b5 =       4.904  ;
c5 =      -2.622 ;
a6 =    -0.02089;
b6 =       5.068  ;
c6 =      0.2548 ;
F_y =   u_VSP*( a1*sin(b1*alpha+c1) + ...
                a2*sin(b2*alpha+c2) + ...
                a3*sin(b3*alpha+c3) + ...
                a4*sin(b4*alpha+c4) + ...
                a5*sin(b5*alpha+c5) + ...
                a6*sin(b6*alpha+c6));

== matlab function CSE1_HIL_full_Test/Controller/CtrlCustom_SLX/Pose/MATLAB Function ==
  data: deg input; rad output
function rad = map_deg2rad(deg)
% maps deg in [-180,180] to rad in (-pi, pi]

rad = deg2rad(deg);

if rad <= -pi
    rad = 2*pi - rad;
elseif rad > pi
    rad = rad - 2*pi;
end

end

== matlab function CSE1_HIL_full_Test/Controller/CtrlCustom_SLX/Oberserver/MATLAB Function ==
  data: x_hat input; psi input; result output; D input; M input
function result = f_A(x_hat, psi, D, M)

% Define the rotation matrix R
R = [
    [cos(psi) -sin(psi) 0];
    [sin(psi) cos(psi) 0];
    [0 0 1]
];

% define system matrix A
A = [
    [zeros(3) R zeros(3)];
    [zeros(3) -M\D M\R'];
    [zeros(3,9)];
];

result = A*x_hat;

== matlab function CSE1_HIL_full_Test/Controller/CtrlCustom_SLX/MATLAB Function ==
  data: eta input; tau output; nu input; eta_d input; eta_d_prime input; eta_d_prime2 input; U_ref input; my input; M input; D input; Kp input; s_dot output size=1; Kd input
function [tau, s_dot]= maneuvering_controller(eta, nu, ...
    eta_d, eta_d_prime, eta_d_prime2, U_ref, my, M, D, Kp, Kd)



%% calculate rotation matrix

psi = eta(3);
R = [
    [cos(psi) -sin(psi) 0];
    [sin(psi) cos(psi) 0];
    [0 0 1]
];

r = nu(3);
S = [
    [0 -r 0];
    [r 0 0];
    [0 0 0];
];


%% Calculate new error in position

z1 = R'*(eta - eta_d);
V1_prime = - z1' * R' * eta_d_prime;


%% Speed assignment

Us = U_ref / norm(eta_d_prime(1:2));
Us_prime = - (norm(eta_d_prime(1:2)'*eta_d_prime2(1:2))*U_ref) / norm(eta_d_prime(1:2))^3; %


%% Update the path variables rate of change

%s_dot = Us - (my / norm(eta_d_prime)) * V1_prime;
s_dot = Us;


%% Calculate control variable terms

% first control variable wrt. path variable
a1_s = Kp*R'*eta_d_prime + R'*eta_d_prime2*Us + R'*eta_d_prime*Us_prime;

% first control variable wrt. time
a1_dot = Kp*S*z1 - Kp*nu - S*R'*eta_d_prime*Us + a1_s*s_dot;

% first control variable
a1 = - Kp*z1 + R'*eta_d_prime*Us;

% error in second step 
z2 = nu - a1;

%% Maneuvering control law

tau = - z1 - Kd*z2 + D*nu + M*a1_dot;

end

== matlab function CSE1_HIL_full_Test/Controller/CtrlCustom_SLX/Oberserver/MATLAB Function1 ==
  data: L1 input; L2 input; L3 input; M input; psi input; eta_diff input; result output
function result = f_L(L1, L2, L3, M, psi, eta_diff)

% Define the rotation matrix R
R = [
    [cos(psi) -sin(psi) 0];
    [sin(psi) cos(psi) 0];
    [0 0 1]
];

L = [L1; M\R'*L2; L3];

result = L*eta_diff;
end

== matlab function CSE1_HIL_full_Test/Controller/CtrlCustom_SLX/Oberserver/MATLAB Function2 ==
  data: previous_measurements input; previous_measurements_new output; eta_measured input; signal_available input; eta_output output; eta_estimated input
function [previous_measurements_new, eta_output] = signal_check(previous_measurements, eta_measured, signal_available, eta_estimated)

if signal_available
    
    % check if signal has stalled
    has_stalled = true;
    for i=1:3
       if eta_measured ~= previous_measurements(i)
           has_stalled = false;
           break
       end
    end
    
    % determine output
    if has_stalled
        eta_output = eta_estimated;
    else
        eta_output = eta_measured;
    end
   
else
   eta_output = eta_estimated; 
end

% update previous measurements
previous_measurements_new = circshift(previous_measurements, 1, 2);
previous_measurements_new(:,1) = eta_measured;
   
end

== matlab function CSE1_HIL_full_Test/Controller/CtrlCustom_SLX/MATLAB Function3 ==
  data: use_elipsoidal_path input; P1 input; P2 input; Pc input; R input; s input; eta_d output; eta_d_prime output; eta_d_prime2 output
function [eta_d, eta_d_prime, eta_d_prime2] = guidance(... 
    use_elipsoidal_path, P1, P2, Pc, R, s)
% elipsoidal_path: when true, the elipsoidal path is used
% P1: start point for straight line path
% P2: end point for straigt line path
% Pc: center point for elipsoidal path
% R: diag(rx,ry) used in radius of elipsoidal path


%% find desired position along path

% eta_d = [x_d, y_d, psi_d]
eta_d = zeros(3,1);
eta_d_prime = zeros(3,1);
eta_d_prime2 = zeros(3,1);
eta_d_prime3 = zeros(3,1);

if use_elipsoidal_path
    eta_d(1:2) = Pc + R * [cos(2*pi*s), sin(2*pi*s)]';
    eta_d_prime(1:2) = 2*pi * R * [-sin(2*pi*s), cos(2*pi*s)]';
    eta_d_prime2(1:2) = 4*pi^2 * R * [-cos(2*pi*s), -sin(2*pi*s)]';
    eta_d_prime3(1:2) = 8*pi^3 * R * [sin(2*pi*s), -cos(2*pi*s)]';
    
else % use straight line path
    eta_d(1:2) = (1 - s) * P1 + s * P2;
    eta_d_prime(1:2) = P2 - P1;
    
end

eta_d(3) = atan2(eta_d_prime(2), eta_d_prime(1)); 
eta_d_prime(3) = (eta_d_prime(1)*eta_d_prime2(2) - ...
    eta_d_prime2(1)*eta_d_prime(2)) / norm(eta_d_prime(1:2))^2;

% psi_d_prime2 is very long
term1 = eta_d_prime3(2)/eta_d_prime(1);
term2 = (eta_d_prime2(2)*eta_d_prime2(1))/(eta_d_prime(1)^2);
term3 = (eta_d_prime(2)*eta_d_prime2(1)^2)/(eta_d_prime(1)^3);
term4 = (eta_d_prime(2)*eta_d_prime3(1))/(eta_d_prime(1)^2);
term5 = (eta_d_prime(2)^2)/(eta_d_prime(1)^2);
term6 = eta_d_prime2(2)/eta_d_prime(1);
term7 = eta_d_prime(2)*eta_d_prime2(1)/eta_d_prime(1)^2;
term8 = eta_d_prime(2)*eta_d_prime2(2)/eta_d_prime(1)^2;
term9 = ((eta_d_prime(2)^2)*eta_d_prime2(1))/((eta_d_prime(1))^3);
term10 = (eta_d_prime(2)^2)/(eta_d_prime(1)^2);
eta_d_prime2(3) = (term1 - 2*term2 + 2*term3 - term4)/(term5 + 1) - ...
    ((term6 - term7)*(2*term8 - 2*term9))/(term10 + 1)^2;


%% Check if the end of the path has been reached


end
